simulink model "matrix6_drive"  (R2018b)
settings: Solver=VariableStepAuto  StartTime=0.0  StopTime=1  RelTol=1e-7
model workspace (MAT data in the model file):
  A1 = 0.212
  A2 = 0.0033
  AMP1 = 0.209333333333
  AMP2 = 0.0330526315789
  B1 = 0.311
  B2 = 0.0075
  C1 = 0.1
  C2 = 0.0084
  Ce1 = 0.27
  Ce2 = 0.12
  Cm1 = 0.36
  Cm2 = 0.12
  D1 = 0.1
  D2 = 0.001
  E1 = 0.1
  E2 = 0.001
  F1 = 0.1
  F2 = 0.001
  Jdrv1 = 7.5e-06
  Jdrv2 = 2.51e-06
  Kf1 = 0.1
  Kf2 = 0.1
  L1 = 0.032
  L2 = 0.0194
  R1 = 0.32
  R2 = 0.485
  RAMP = 0.209333333333
  T1 = 0.05
  T2 = 0.0001
  Tpwm = 6.25e-05
  Umax = 27
  Xc2 = 0
  Yc2 = 0.0148
  a = 0
  b = -2.09439510239
  c = 2.09439510239
  dt1 = 0.6
  dt2 = 0.6
  dx1 = 3.14
  dx2 = 1.57
  g = 9.81
  m2 = 1.13085
  omega1 = 1.005
  omega2 = 6.28
  poles = 8
libraries: simulink x1
(part 1 of 2)
settings Model: Creator=Sainquake  LastModifiedBy=Sainquake

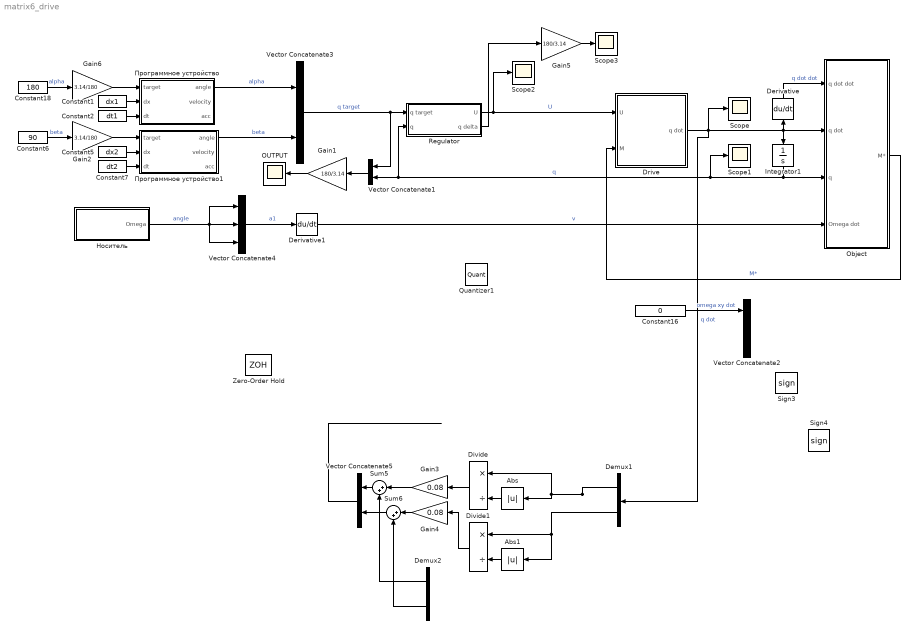
== system matrix6_drive ==
  Abs : Abs  ZeroCross=off
  Abs1 : Abs  ZeroCross=off
  Constant1 : Constant  Value=dx1
  Constant16 : Constant  Value=0
  Constant18 : Constant  Value=180
  Constant2 : Constant  Value=dt1
  Constant5 : Constant  Value=dx2
  Constant6 : Constant  Value=90
  Constant7 : Constant  Value=dt2
  Demux1 : Demux  Outputs=2
  Demux2 : Demux  Outputs=2
  Derivative : Derivative
  Derivative1 : Derivative
  Divide : Product  Inputs=*/
  Divide1 : Product  Inputs=*/
  Drive : Subsystem
  Gain1 : Gain  Gain=180/3.14
  Gain2 : Gain  Gain=3.14/180
  Gain3 : Gain  Gain=0.08
  Gain4 : Gain  Gain=0.08
  Gain5 : Gain  Gain=180/3.14
  Gain6 : Gain  Gain=3.14/180
  Integrator1 : Integrator
  OUTPUT : Scope
  Object : Subsystem
  Quantizer1 : Quantizer  QuantizationInterval=0.0003
  Regulator : Subsystem
  Scope{,1..3} (4 alike) : Scope
  Sign3 : Signum  ZeroCross=off
  Sign4 : Signum  ZeroCross=off
  Sum5 : Sum  Inputs=|++
  Sum6 : Sum  Inputs=|++
  Vector Concatenate1 : Concatenate
  Vector Concatenate2 : Concatenate  NumInputs=3
  Vector Concatenate3 : Concatenate
  Vector Concatenate4 : Concatenate  NumInputs=3
  Vector Concatenate5 : Concatenate
  Zero-Order Hold : ZeroOrderHold  SampleTime=Tpwm
  Носитель : Subsystem
  Программное устройство : Subsystem
  Программное устройство1 : Subsystem
  wires:
  Integrator1/1 -> Regulator/2(q), Vector Concatenate1/2, Scope1/1, Object/3("q ")  "q"
  ? -> Vector Concatenate2/3  "omega zy dot"
  ? -> Vector Concatenate2/2  "omega yy dot"
  Constant16/1 -> Vector Concatenate2/1  "omega xy dot"
  Программное устройство1/1(angle) -> Vector Concatenate3/2  "beta"
  Программное устройство/1(angle) -> Vector Concatenate3/1  "alpha"
  Drive/1(q dot) -> Demux1/1, Integrator1/1, Object/2(q dot), Derivative/1, Scope/1  "q dot"
  Object/1(M*) -> Drive/2(M)  "M*"
  Regulator/1("U ") -> Scope2/1, Drive/1(U)  "U"
  Divide/1 -> Gain3/1
  Divide1/1 -> Gain4/1
  Vector Concatenate5/1 -> ?
  Gain3/1 -> Sum5/1
  Demux2/1 -> Sum5/2
  Gain4/1 -> Sum6/1
  Demux2/2 -> Sum6/2
  Sum5/1 -> Vector Concatenate5/1
  Sum6/1 -> Vector Concatenate5/2
  Derivative/1 -> Object/1(q dot dot)  "q dot dot"
  Vector Concatenate3/1 -> Vector Concatenate1/1, Regulator/1(q target)  "q target"
  Vector Concatenate1/1 -> Gain1/1
  Gain1/1 -> OUTPUT/1
  Constant2/1 -> Программное устройство/3(dt)
  Gain6/1 -> Программное устройство/1(target)
  Constant1/1 -> Программное устройство/2("dx ")
  Constant18/1 -> Gain6/1  "alpha"
  Constant6/1 -> Gain2/1  "beta"
  Gain2/1 -> Программное устройство1/1(target)
  Constant7/1 -> Программное устройство1/3(dt)
  Constant5/1 -> Программное устройство1/2("dx ")
  Regulator/2(q delta) -> Gain5/1
  Gain5/1 -> Scope3/1
  Abs/1 -> Divide/2
  Demux1/1 -> Divide/1, Abs/1
  Abs1/1 -> Divide1/2
  Demux1/2 -> Abs1/1, Divide1/1
  Vector Concatenate4/1 -> Derivative1/1  "a1"
  Носитель/1(Omega) -> Vector Concatenate4/3, Vector Concatenate4/1, Vector Concatenate4/2  "angle"
  Derivative1/1 -> Object/4(Omega dot)  "v"

== system matrix6_drive/Drive ==
  U : Inport
  M : Inport  Port=2
  Demux : Demux  Outputs=2
  Demux1 : Demux  Outputs=2
  Scope : Scope
  Sum : Sum  Inputs=|+-
  Sum1 : Sum  Inputs=-+|
  Transfer Fcn : TransferFcn  Numerator=[Cm1]  Denominator=[L1 R1]
  Transfer Fcn1 : TransferFcn  Numerator=1  Denominator=[Cm1*Ce1]
  Transfer Fcn2 : TransferFcn  Numerator=[L1 R1]  Denominator=[0.0001 1]
  Transfer Fcn3 : TransferFcn  Numerator=[Cm2]  Denominator=[L2 R2]
  Transfer Fcn4 : TransferFcn  Numerator=1  Denominator=[Cm2*Ce2]
  Transfer Fcn5 : TransferFcn  Numerator=[L2 R2]  Denominator=[0.0001 1]
  Vector Concatenate6 : Concatenate
  Привод : Subsystem
  Привод1 : Subsystem
  q dot : Outport
  wires:
  Sum/1 -> Transfer Fcn2/1
  Transfer Fcn3/1 -> Sum1/2
  Demux1/2 -> Sum1/1
  Demux/1 -> Привод/1(U)
  Vector Concatenate6/1 -> q dot/1, Scope/1  "a1"
  Transfer Fcn/1 -> Sum/1
  Transfer Fcn5/1 -> Transfer Fcn4/1
  Transfer Fcn2/1 -> Transfer Fcn1/1
  Demux1/1 -> Привод/2(M load)
  Demux/2 -> Transfer Fcn3/1
  Sum1/1 -> Transfer Fcn5/1
  Transfer Fcn1/1 -> ?
  Transfer Fcn4/1 -> Vector Concatenate6/2
  U/1 -> Demux/1
  M/1 -> Demux1/1
  Привод/2(velocity) -> Vector Concatenate6/1
  Привод1/2(velocity) -> ?

== system matrix6_drive/Object ==
  q dot dot : Inport
  q dot : Inport  Port=2
  "q " : Inport  Port=3
  Omega dot : Inport  Port=4
  A(q) : Subsystem
  B(t,q) : Subsystem
  F(q,q dot) : Subsystem
  Integrator2 : Integrator
  Matrix Multiply1 : Product  Multiplication=Matrix(*)
  Matrix Multiply2 : Product  Multiplication=Matrix(*)
  Q*(t,q) : Subsystem
  Sum : Sum  Inputs=+++
  Sum1 : Sum  Inputs=+++
  W(t,q) : Subsystem
  M* : Outport
  wires:
  Integrator2/1 -> B(t,q)/1(omega), W(t,q)/1(Omega)
  Sum1/1 -> M*/1  "M*"
  A(q)/1(A) -> Matrix Multiply1/1
  q dot dot/1 -> Matrix Multiply1/2  "q dot dot"
  Omega dot/1 -> Integrator2/1, W(t,q)/2(Omega dot)  "a1"
  Sum/1 -> Sum1/1
  Matrix Multiply1/1 -> Sum/1
  Matrix Multiply2/1 -> Sum/2
  B(t,q)/1(B) -> Matrix Multiply2/1
  q dot/1 -> F(q,q dot)/1(q dot), Matrix Multiply2/2  "q dot"
  "q "/1 -> F(q,q dot)/2(q), B(t,q)/2(q), A(q)/1(q), Q*(t,q)/1(q), W(t,q)/3(q)  "q"
  W(t,q)/1(W) -> Sum1/2
  Q*(t,q)/1(Q) -> Sum1/3
  F(q,q dot)/1(F(q,q dot)) -> Sum/3

== system matrix6_drive/Regulator ==
  q target : Inport
  q : Inport  Port=2
  Demux : Demux  Outputs=2
  Demux3 : Demux  Outputs=2
  Gain2 : Gain  Gain=700
  Gain5 : Gain  Gain=300
  Saturation : Saturate  UpperLimit=27  LowerLimit=-27  ZeroCross=off
  Saturation1 : Saturate  UpperLimit=27  LowerLimit=-27  ZeroCross=off
  Sum2 : Sum  Inputs=|+-
  Sum3 : Sum  Inputs=|+-
  Transfer Fcn : TransferFcn  Numerator=[T1 1]  Denominator=[T2 1]
  Transfer Fcn1 : TransferFcn  Numerator=[0.05 1]  Denominator=[0.0005 1]
  Vector Concatenate1 : Concatenate
  Vector Concatenate2 : Concatenate
  "U " : Outport
  q delta : Outport  Port=2
  wires:
  Demux/1 -> Sum3/2
  Demux/2 -> Sum2/2
  Sum3/1 -> Vector Concatenate2/1, Gain2/1
  Transfer Fcn1/1 -> Vector Concatenate1/2
  Sum2/1 -> Vector Concatenate2/2, Gain5/1
  Transfer Fcn/1 -> Vector Concatenate1/1
  Demux3/2 -> Sum2/1
  Gain2/1 -> Transfer Fcn/1
  q target/1 -> Demux3/1  "q target"
  Gain5/1 -> Transfer Fcn1/1
  Demux3/1 -> Sum3/1
  q/1 -> Demux/1  "q"
  Vector Concatenate1/1 -> "U "/1  "U"
  Vector Concatenate2/1 -> q delta/1  "U"

== system matrix6_drive/Носитель ==
  Clock : Clock
  Gain : Gain  Gain=AMP1
  Gain1 : Gain  Gain=AMP2
  Gain2 : Gain  Gain=omega1
  Gain3 : Gain  Gain=omega2
  Ramp : simulink/Sources/Ramp  slope=RAMP  start=0  InitialOutput=0
  Sum1 : Sum  Inputs=+++
  Trigonometric Function : Trigonometry
  Trigonometric Function1 : Trigonometry
  Omega : Outport
  wires:
  Trigonometric Function/1 -> Gain/1
  Trigonometric Function1/1 -> Gain1/1
  Clock/1 -> Gain2/1, Gain3/1
  Gain2/1 -> Trigonometric Function/1
  Gain3/1 -> Trigonometric Function1/1
  Gain/1 -> Sum1/2
  Gain1/1 -> Sum1/3
  Sum1/1 -> Omega/1
  Ramp/1 -> Sum1/1

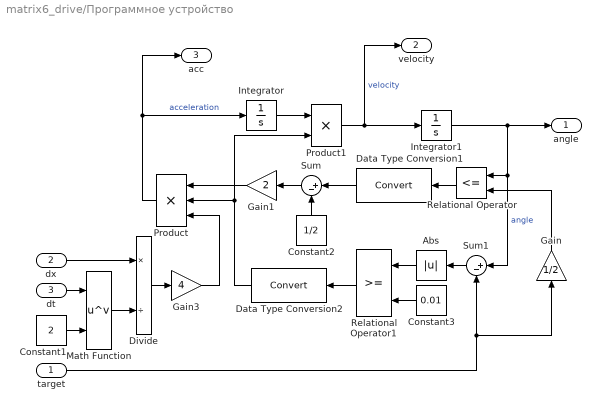
== system matrix6_drive/Программное устройство ==
  target : Inport
  "dx " : Inport  Port=2
  dt : Inport  Port=3
  Abs : Abs  ZeroCross=off
  Constant1 : Constant  Value=2
  Constant2 : Constant  Value=1/2
  Constant3 : Constant  Value=0.01
  Data Type Conversion1 : DataTypeConversion
  Data Type Conversion2 : DataTypeConversion
  Divide : Product  Inputs=*/
  Gain : Gain  Gain=1/2
  Gain1 : Gain  Gain=2
  Gain3 : Gain  Gain=4
  Integrator : Integrator
  Integrator1 : Integrator
  Math Function : Math  Operator=pow  SaturateOnIntegerOverflow=on
  Product : Product  Inputs=3
  Product1 : Product
  Relational Operator : RelationalOperator  Operator=<=  OutDataTypeStr=boolean  ZeroCross=off  RndMeth=Simplest
  Relational Operator1 : RelationalOperator  OutDataTypeStr=boolean  ZeroCross=off  RndMeth=Simplest
  Sum : Sum  Inputs=|+-
  Sum1 : Sum  Inputs=|+-
  angle : Outport
  velocity : Outport  Port=2
  acc : Outport  Port=3
  wires:
  "dx "/1 -> Divide/1
  Constant1/1 -> Math Function/2
  Gain3/1 -> Product/3
  Data Type Conversion1/1 -> Sum/1
  Sum/1 -> Gain1/1
  Product/1 -> Integrator/1, acc/1  "acceleration"
  Product1/1 -> Integrator1/1, velocity/1  "velocity"
  Abs/1 -> Relational Operator1/1
  Relational Operator1/1 -> Data Type Conversion2/1
  Sum1/1 -> Abs/1
  Data Type Conversion2/1 -> Product1/2, Product/2
  Divide/1 -> Gain3/1
  Constant2/1 -> Sum/2
  Integrator/1 -> Product1/1
  target/1 -> Gain/1, Sum1/2
  Math Function/1 -> Divide/2
  Gain/1 -> Relational Operator/2
  Gain1/1 -> Product/1
  Relational Operator/1 -> Data Type Conversion1/1
  dt/1 -> Math Function/1
  Constant3/1 -> Relational Operator1/2
  Integrator1/1 -> angle/1, Sum1/1, Relational Operator/1  "angle"

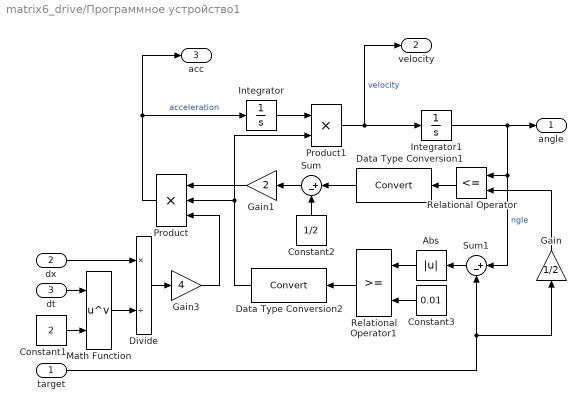
== system matrix6_drive/Программное устройство1 ==
  target : Inport
  "dx " : Inport  Port=2
  dt : Inport  Port=3
  Abs : Abs  ZeroCross=off
  Constant1 : Constant  Value=2
  Constant2 : Constant  Value=1/2
  Constant3 : Constant  Value=0.01
  Data Type Conversion1 : DataTypeConversion
  Data Type Conversion2 : DataTypeConversion
  Divide : Product  Inputs=*/
  Gain : Gain  Gain=1/2
  Gain1 : Gain  Gain=2
  Gain3 : Gain  Gain=4
  Integrator : Integrator
  Integrator1 : Integrator
  Math Function : Math  Operator=pow  SaturateOnIntegerOverflow=on
  Product : Product  Inputs=3
  Product1 : Product
  Relational Operator : RelationalOperator  Operator=<=  OutDataTypeStr=boolean  ZeroCross=off  RndMeth=Simplest
  Relational Operator1 : RelationalOperator  OutDataTypeStr=boolean  ZeroCross=off  RndMeth=Simplest
  Sum : Sum  Inputs=|+-
  Sum1 : Sum  Inputs=|+-
  angle : Outport
  velocity : Outport  Port=2
  acc : Outport  Port=3
  wires:
  "dx "/1 -> Divide/1
  Constant1/1 -> Math Function/2
  Gain3/1 -> Product/3
  Data Type Conversion1/1 -> Sum/1
  Sum/1 -> Gain1/1
  Product/1 -> Integrator/1, acc/1  "acceleration"
  Product1/1 -> Integrator1/1, velocity/1  "velocity"
  Abs/1 -> Relational Operator1/1
  Relational Operator1/1 -> Data Type Conversion2/1
  Sum1/1 -> Abs/1
  Data Type Conversion2/1 -> Product1/2, Product/2
  Divide/1 -> Gain3/1
  Constant2/1 -> Sum/2
  Integrator/1 -> Product1/1
  target/1 -> Gain/1, Sum1/2
  Math Function/1 -> Divide/2
  Gain/1 -> Relational Operator/2
  Gain1/1 -> Product/1
  Relational Operator/1 -> Data Type Conversion1/1
  dt/1 -> Math Function/1
  Constant3/1 -> Relational Operator1/2
  Integrator1/1 -> angle/1, Sum1/1, Relational Operator/1  "ngle"

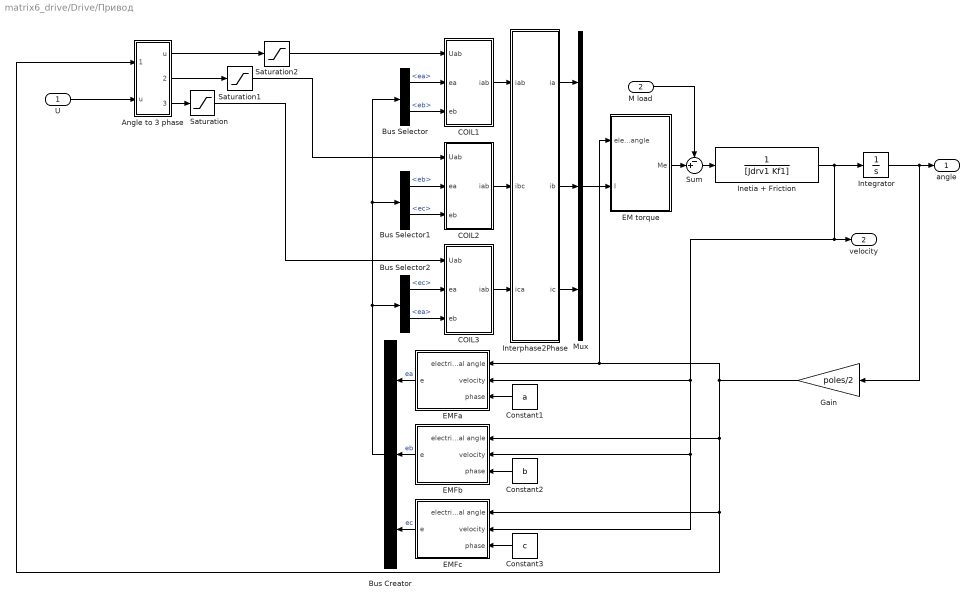
== system matrix6_drive/Drive/Привод ==
  U : Inport
  M load : Inport  Port=2
  Angle to 3 phase : Subsystem
  Bus Creator : BusCreator  Inputs=3
  Bus Selector : BusSelector  OutputSignals=ea,eb
  Bus Selector1 : BusSelector  OutputSignals=eb,ec
  Bus Selector2 : BusSelector  OutputSignals=ec,ea
  COIL1 : Subsystem
  "COIL2 " : Subsystem
  COIL3 : Subsystem
  Constant1 : Constant  Value=a
  Constant2 : Constant  Value=b
  Constant3 : Constant  Value=c
  EM torque : Subsystem
  EMFa : Subsystem
  EMFb : Subsystem
  EMFc : Subsystem
  Gain : Gain  Gain=poles/2
  Inetia + Friction : TransferFcn  Denominator=[Jdrv1 Kf1]
  Integrator : Integrator
  Interphase2Phase : Subsystem
  Mux : Mux  Inputs=3
  Saturation : Saturate  UpperLimit=Umax  LowerLimit=0  ZeroCross=off
  Saturation1 : Saturate  UpperLimit=Umax  LowerLimit=0  ZeroCross=off
  Saturation2 : Saturate  UpperLimit=Umax  LowerLimit=0  ZeroCross=off
  Sum : Sum  Inputs=-+|
  angle : Outport
  velocity : Outport  Port=2
  wires:
  M load/1 -> Sum/1
  Bus Creator/1 -> Bus Selector/1, Bus Selector1/1, Bus Selector2/1
  COIL1/1(iab) -> Interphase2Phase/1(iab)
  Interphase2Phase/1(ia) -> Mux/1
  Bus Selector2/2 -> COIL3/3(eb)  "<ea>"
  Gain/1 -> Angle to 3 phase/1(target), EMFc/1(electrical angle), EMFb/1(electrical angle), EM torque/1(electrical angle), EMFa/1(electrical angle)
  Bus Selector2/1 -> COIL3/2("ea ")  "<ec>"
  Bus Selector1/1 -> "COIL2 "/2("ea ")  "<eb>"
  Bus Selector1/2 -> "COIL2 "/3(eb)  "<ec>"
  Mux/1 -> EM torque/2(I)
  Bus Selector/2 -> COIL1/3(eb)  "<eb>"
  Bus Selector/1 -> COIL1/2("ea ")  "<ea>"
  Sum/1 -> Inetia + Friction/1
  Constant2/1 -> EMFb/3(phase)
  Constant3/1 -> EMFc/3(phase)
  Constant1/1 -> EMFa/3(phase)
  Inetia + Friction/1 -> Integrator/1, velocity/1, EMFc/2(velocity), EMFb/2(velocity), EMFa/2(velocity)
  EMFa/1(e) -> Bus Creator/1  "ea"
  EMFc/1(e) -> Bus Creator/3  "ec"
  EM torque/1(Me) -> Sum/2
  Interphase2Phase/3(ic) -> Mux/3
  "COIL2 "/1(iab) -> Interphase2Phase/2("ibc ")
  Angle to 3 phase/1("u ") -> Saturation2/1
  EMFb/1(e) -> Bus Creator/2  "eb"
  Angle to 3 phase/3(u 2) -> Saturation/1
  Angle to 3 phase/2(u 1) -> Saturation1/1
  Interphase2Phase/2(ib) -> Mux/2
  COIL3/1(iab) -> Interphase2Phase/3(ica)
  U/1 -> Angle to 3 phase/2(u)
  Integrator/1 -> Gain/1, angle/1
  Saturation2/1 -> COIL1/1(Uab)
  Saturation1/1 -> "COIL2 "/1(Uab)
  Saturation/1 -> COIL3/1(Uab)

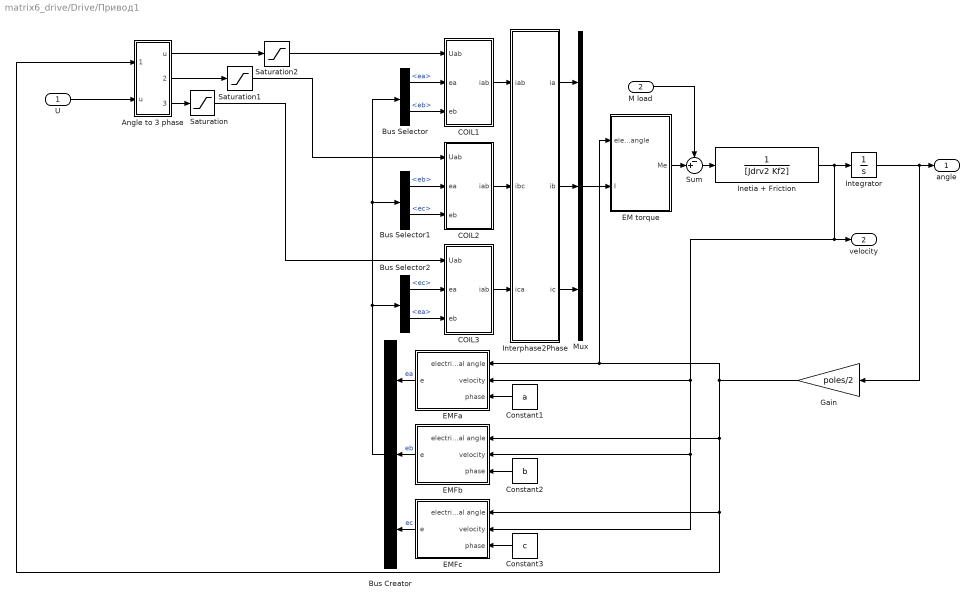
== system matrix6_drive/Drive/Привод1 ==
  U : Inport
  M load : Inport  Port=2
  Angle to 3 phase : Subsystem
  Bus Creator : BusCreator  Inputs=3
  Bus Selector : BusSelector  OutputSignals=ea,eb
  Bus Selector1 : BusSelector  OutputSignals=eb,ec
  Bus Selector2 : BusSelector  OutputSignals=ec,ea
  COIL1 : Subsystem
  "COIL2 " : Subsystem
  COIL3 : Subsystem
  Constant1 : Constant  Value=a
  Constant2 : Constant  Value=b
  Constant3 : Constant  Value=c
  EM torque : Subsystem
  EMFa : Subsystem
  EMFb : Subsystem
  EMFc : Subsystem
  Gain : Gain  Gain=poles/2
  Inetia + Friction : TransferFcn  Denominator=[Jdrv2 Kf2]
  Integrator : Integrator
  Interphase2Phase : Subsystem
  Mux : Mux  Inputs=3
  Saturation : Saturate  UpperLimit=Umax  LowerLimit=0  ZeroCross=off
  Saturation1 : Saturate  UpperLimit=Umax  LowerLimit=0  ZeroCross=off
  Saturation2 : Saturate  UpperLimit=Umax  LowerLimit=0  ZeroCross=off
  Sum : Sum  Inputs=-+|
  angle : Outport
  velocity : Outport  Port=2
  wires:
  Saturation/1 -> COIL3/1(Uab)
  Saturation1/1 -> "COIL2 "/1(Uab)
  Saturation2/1 -> COIL1/1(Uab)
  Integrator/1 -> Gain/1, angle/1
  U/1 -> Angle to 3 phase/2(u)
  COIL3/1(iab) -> Interphase2Phase/3(ica)
  Interphase2Phase/2(ib) -> Mux/2
  Angle to 3 phase/2(u 1) -> Saturation1/1
  Angle to 3 phase/3(u 2) -> Saturation/1
  EMFb/1(e) -> Bus Creator/2  "eb"
  Angle to 3 phase/1("u ") -> Saturation2/1
  "COIL2 "/1(iab) -> Interphase2Phase/2("ibc ")
  Interphase2Phase/3(ic) -> Mux/3
  EM torque/1(Me) -> Sum/2
  EMFc/1(e) -> Bus Creator/3  "ec"
  EMFa/1(e) -> Bus Creator/1  "ea"
  Inetia + Friction/1 -> Integrator/1, EMFa/2(velocity), EMFb/2(velocity), EMFc/2(velocity), velocity/1
  Constant1/1 -> EMFa/3(phase)
  Constant3/1 -> EMFc/3(phase)
  Constant2/1 -> EMFb/3(phase)
  Sum/1 -> Inetia + Friction/1
  Bus Selector/1 -> COIL1/2("ea ")  "<ea>"
  Bus Selector/2 -> COIL1/3(eb)  "<eb>"
  Mux/1 -> EM torque/2(I)
  Bus Selector1/2 -> "COIL2 "/3(eb)  "<ec>"
  Bus Selector1/1 -> "COIL2 "/2("ea ")  "<eb>"
  Bus Selector2/1 -> COIL3/2("ea ")  "<ec>"
  Gain/1 -> EMFa/1(electrical angle), EM torque/1(electrical angle), EMFb/1(electrical angle), EMFc/1(electrical angle), Angle to 3 phase/1(target)
  Bus Selector2/2 -> COIL3/3(eb)  "<ea>"
  Interphase2Phase/1(ia) -> Mux/1
  COIL1/1(iab) -> Interphase2Phase/1(iab)
  Bus Creator/1 -> Bus Selector2/1, Bus Selector1/1, Bus Selector/1
  M load/1 -> Sum/1

== system matrix6_drive/Object/A(q) ==
  q : Inport
  B(beta) : Subsystem
  Constant10 : Constant  Value=C2
  Constant7 : Constant  Value=B1
  D(beta) : Subsystem
  Demux : Demux  Outputs=2
  Display5 : Display
  Gain : Gain  Gain=-1
  Sum : Sum  Inputs=|++
  Vector Concatenate1 : Concatenate
  Vector Concatenate2 : Concatenate
  Vector Concatenate6 : Concatenate  Mode=Multidimensional array  ConcatenateDimension=2
  A : Outport
  wires:
  q/1 -> Demux/1
  Constant7/1 -> Sum/2
  Vector Concatenate2/1 -> Vector Concatenate6/2  "a2"
  Sum/1 -> Vector Concatenate1/1  "a11"
  Constant10/1 -> Vector Concatenate2/2  "a22"
  Vector Concatenate1/1 -> Vector Concatenate6/1  "a1"
  B(beta)/1(B) -> Sum/1
  D(beta)/1(D) -> Gain/1
  Vector Concatenate6/1 -> A/1, Display5/1  "A"
  Gain/1 -> Vector Concatenate1/2, Vector Concatenate2/1  "a12"
  Demux/2 -> B(beta)/1(beta), D(beta)/1(beta)

== system matrix6_drive/Object/B(t,q) ==
  omega : Inport
  q : Inport  Port=2
  Constant : Constant  Value=0
  Gain : Gain  Gain=-1
  Vector Concatenate3 : Concatenate
  Vector Concatenate4 : Concatenate
  Vector Concatenate5 : Concatenate  Mode=Multidimensional array  ConcatenateDimension=2
  b(t,alpha,beta) : Subsystem
  B : Outport
  wires:
  Vector Concatenate3/1 -> Vector Concatenate5/1  "a1"
  Vector Concatenate5/1 -> B/1  "A"
  Vector Concatenate4/1 -> Vector Concatenate5/2  "a2"
  b(t,alpha,beta)/1(b) -> Vector Concatenate3/2, Gain/1
  Gain/1 -> Vector Concatenate4/1
  Constant/1 -> Vector Concatenate4/2, Vector Concatenate3/1
  omega/1 -> b(t,alpha,beta)/1(omega)
  q/1 -> b(t,alpha,beta)/2(q)

== system matrix6_drive/Object/F(q,q dot) ==
  q dot : Inport
  q : Inport  Port=2
  Constant : Constant  Value=2
  Constant1 : Constant  Value=2
  Demux : Demux  Outputs=2
  Demux1 : Demux  Outputs=2
  E(beta) : Subsystem
  F(alpha,beta) : Subsystem
  F(beta) : Subsystem
  Gain : Gain  Gain=2
  Math Function : Math  Operator=pow  SaturateOnIntegerOverflow=on
  Math Function1 : Math  Operator=pow  SaturateOnIntegerOverflow=on
  Product : Product  Inputs=3
  Product1 : Product
  Product2 : Product
  Sum : Sum  Inputs=|--
  Vector Concatenate : Concatenate
  F(q,q dot) : Outport
  wires:
  q dot/1 -> Demux/1
  Product/1 -> Gain/1
  Demux/2 -> Product/2, Math Function/1  "beta dot"
  F(alpha,beta)/1(F(q)) -> Product/3
  q/1 -> Demux1/1, F(alpha,beta)/1(q)
  Constant/1 -> Math Function/2
  Math Function/1 -> Product1/1
  E(beta)/1(E) -> Product1/2
  Demux1/2 -> E(beta)/1(beta), F(beta)/1(beta)
  Gain/1 -> Sum/1
  Product1/1 -> Sum/2
  Constant1/1 -> Math Function1/2
  Demux/1 -> Product/1, Math Function1/1  "alpha dot"
  Math Function1/1 -> Product2/2
  F(beta)/1(F) -> Product2/1
  Product2/1 -> Vector Concatenate/2
  Sum/1 -> Vector Concatenate/1
  Vector Concatenate/1 -> F(q,q dot)/1

== system matrix6_drive/Object/Q*(t,q) ==
  q : Inport
  Constant : Constant  Value=0
  Constant1 : Constant  Value=m2
  Constant2 : Constant  Value=Xc2
  Constant3 : Constant  Value=Yc2
  Demux : Demux  Outputs=2
  Gain : Gain  Gain=g
  Product : Product
  Product1 : Product
  Product2 : Product
  Sum : Sum  Inputs=+-
  Trigonometric Function : Trigonometry  Operator=cos
  Trigonometric Function1 : Trigonometry
  Vector Concatenate1 : Concatenate
  Q : Outport
  wires:
  Vector Concatenate1/1 -> Q/1  "q"
  Constant/1 -> Vector Concatenate1/1
  Product/1 -> Vector Concatenate1/2
  Gain/1 -> Product/1
  Constant1/1 -> Gain/1
  q/1 -> Demux/1
  Trigonometric Function/1 -> Product1/1
  Constant2/1 -> Product1/2
  Product1/1 -> Sum/1
  Constant3/1 -> Product2/2
  Demux/2 -> Trigonometric Function1/1, Trigonometric Function/1  "beta"
  Product2/1 -> Sum/2
  Trigonometric Function1/1 -> Product2/1
  Sum/1 -> Product/2

== system matrix6_drive/Object/W(t,q) ==
  Omega : Inport
  Omega dot : Inport  Port=2
  q : Inport  Port=3
  Vector Concatenate : Concatenate
  "w alpha (t, q) " : Subsystem
  "w beta (t, q)" : Subsystem
  W : Outport
  wires:
  Omega/1 -> "w beta (t, q)"/1(Omega), "w alpha (t, q) "/1(Omega)
  Omega dot/1 -> "w beta (t, q)"/2(Omega dot), "w alpha (t, q) "/2(Omega dot)
  q/1 -> "w beta (t, q)"/3(q), "w alpha (t, q) "/3(q)
  "w alpha (t, q) "/1(w alpha) -> Vector Concatenate/1
  "w beta (t, q)"/1(w alpha) -> Vector Concatenate/2
  Vector Concatenate/1 -> W/1

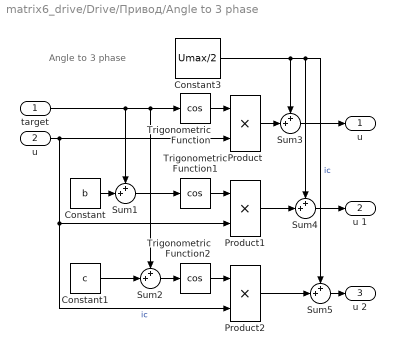
== system matrix6_drive/Drive/Привод/Angle to 3 phase ==
  note: Angle to 3 phase
  target : Inport
  u : Inport  Port=2
  Constant : Constant  Value=b
  Constant1 : Constant  Value=c
  Constant3 : Constant  Value=Umax/2
  Product : Product
  Product1 : Product
  Product2 : Product
  Sum{1..5} (5 alike) : Sum  Inputs=++|
  Trigonometric Function : Trigonometry  Operator=cos
  Trigonometric Function1 : Trigonometry  Operator=cos
  Trigonometric Function2 : Trigonometry  Operator=cos
  "u " : Outport
  u 1 : Outport  Port=2
  u 2 : Outport  Port=3
  wires:
  Sum3/1 -> "u "/1
  target/1 -> Sum2/1, Trigonometric Function/1, Sum1/1
  Trigonometric Function2/1 -> Product2/1
  Sum2/1 -> Trigonometric Function2/1
  Trigonometric Function1/1 -> Product1/1
  u/1 -> Product/2, Product2/2, Product1/2  "ic"
  Constant1/1 -> Sum2/2
  Sum1/1 -> Trigonometric Function1/1
  Constant/1 -> Sum1/2
  Trigonometric Function/1 -> Product/1
  Constant3/1 -> Sum5/1, Sum4/1, Sum3/1  "ic"
  Product/1 -> Sum3/2
  Product1/1 -> Sum4/2
  Product2/1 -> Sum5/2
  Sum5/1 -> u 2/1
  Sum4/1 -> u 1/1

== system matrix6_drive/Drive/Привод/COIL1 ==
  note: COILx
  Uab : Inport
  "ea " : Inport  Port=2
  eb : Inport  Port=3
  Sum : Sum  Inputs=|+-
  Sum1 : Sum  Inputs=|+-
  Transfer Fcn : TransferFcn  Denominator=[L1 R1]
  iab : Outport
  wires:
  Uab/1 -> Sum/1
  Transfer Fcn/1 -> iab/1
  Sum/1 -> Transfer Fcn/1
  "ea "/1 -> Sum1/1
  eb/1 -> Sum1/2
  Sum1/1 -> Sum/2

== system matrix6_drive/Drive/Привод/COIL2  ==
  Uab : Inport
  "ea " : Inport  Port=2
  eb : Inport  Port=3
  Sum : Sum  Inputs=|+-
  Sum1 : Sum  Inputs=|+-
  Transfer Fcn : TransferFcn  Denominator=[L1 R1]
  iab : Outport
  wires:
  Uab/1 -> Sum/1
  Transfer Fcn/1 -> iab/1
  Sum/1 -> Transfer Fcn/1
  "ea "/1 -> Sum1/1
  eb/1 -> Sum1/2
  Sum1/1 -> Sum/2

== system matrix6_drive/Drive/Привод/COIL3 ==
  Uab : Inport
  "ea " : Inport  Port=2
  eb : Inport  Port=3
  Sum : Sum  Inputs=|+-
  Sum1 : Sum  Inputs=|+-
  Transfer Fcn : TransferFcn  Denominator=[L1 R1]
  iab : Outport
  wires:
  Uab/1 -> Sum/1
  Transfer Fcn/1 -> iab/1
  Sum/1 -> Transfer Fcn/1
  "ea "/1 -> Sum1/1
  eb/1 -> Sum1/2
  Sum1/1 -> Sum/2

== system matrix6_drive/Drive/Привод/EM torque ==
  note: Electromagnetic Torque
  electrical angle : Inport
  I : Inport  Port=2
  Constant2 : Constant  Value=a
  Constant3 : Constant  Value=b
  Constant4 : Constant  Value=c
  Demux : Demux  Outputs=3
  Gain : Gain  Gain=Cm1
  Product3 : Product
  Product4 : Product
  Product5 : Product
  Subsystem : Subsystem
  Subsystem1 : Subsystem
  Subsystem2 : Subsystem
  Sum : Sum  Inputs=+++
  Me : Outport
  wires:
  Sum/1 -> Gain/1
  Gain/1 -> Me/1
  I/1 -> Demux/1
  Constant2/1 -> Subsystem/2(phase)
  electrical angle/1 -> Subsystem2/1(electrical angle), Subsystem1/1(electrical angle), Subsystem/1(electrical angle)
  Constant3/1 -> Subsystem1/2(phase)
  Constant4/1 -> Subsystem2/2(phase)
  Demux/1 -> Product3/2  "ia"
  Subsystem/1(Out1) -> Product3/1
  Demux/2 -> Product4/2  "ib"
  Demux/3 -> Product5/2  "ic"
  Subsystem1/1(Out1) -> Product4/1
  Subsystem2/1(Out1) -> Product5/1
  Product4/1 -> Sum/2
  Product3/1 -> Sum/1
  Product5/1 -> Sum/3

== system matrix6_drive/Drive/Привод/EMFa ==
  note: EMF
  electrical angle : Inport
  velocity : Inport  Port=2
  phase : Inport  Port=3
  Gain : Gain  Gain=Ce1
  Product1 : Product
  Subsystem : Subsystem
  e : Outport
  wires:
  Gain/1 -> Product1/2
  Product1/1 -> e/1
  velocity/1 -> Gain/1
  phase/1 -> Subsystem/2(phase)
  electrical angle/1 -> Subsystem/1(electrical angle)
  Subsystem/1(Out1) -> Product1/1

== system matrix6_drive/Drive/Привод/EMFb ==
  electrical angle : Inport
  velocity : Inport  Port=2
  phase : Inport  Port=3
  Gain : Gain  Gain=Ce1
  Product1 : Product
  Sum1 : Sum  Inputs=++|
  Trigonometric Function1 : Trigonometry  Operator=cos
  e : Outport
  wires:
  Trigonometric Function1/1 -> Product1/1
  Gain/1 -> Product1/2
  Sum1/1 -> Trigonometric Function1/1
  phase/1 -> Sum1/2
  electrical angle/1 -> Sum1/1
  Product1/1 -> e/1
  velocity/1 -> Gain/1

== system matrix6_drive/Drive/Привод/EMFc ==
  electrical angle : Inport
  velocity : Inport  Port=2
  phase : Inport  Port=3
  Gain : Gain  Gain=Ce1
  Product1 : Product
  Sum1 : Sum  Inputs=++|
  Trigonometric Function1 : Trigonometry  Operator=cos
  e : Outport
  wires:
  Trigonometric Function1/1 -> Product1/1
  Gain/1 -> Product1/2
  Sum1/1 -> Trigonometric Function1/1
  phase/1 -> Sum1/2
  electrical angle/1 -> Sum1/1
  Product1/1 -> e/1
  velocity/1 -> Gain/1

== system matrix6_drive/Drive/Привод/Interphase2Phase ==
  note: Interphase to phase currents
  iab : Inport
  "ibc " : Inport  Port=2
  ica : Inport  Port=3
  Gain : Gain  Gain=1/2
  Gain1 : Gain  Gain=1/2
  Gain2 : Gain  Gain=1/2
  Sum : Sum  Inputs=+--
  Sum1 : Sum  Inputs=+--
  Sum2 : Sum  Inputs=+--
  ia : Outport
  ib : Outport  Port=2
  ic : Outport  Port=3
  wires:
  Gain/1 -> ia/1
  Gain1/1 -> ib/1
  Gain2/1 -> ic/1
  iab/1 -> Sum2/3, Sum1/3, Sum/1
  "ibc "/1 -> Sum2/2, Sum1/1, Sum/2
  ica/1 -> Sum/3, Sum2/1, Sum1/2
  Sum/1 -> Gain/1
  Sum1/1 -> Gain1/1
  Sum2/1 -> Gain2/1

== system matrix6_drive/Drive/Привод1/Angle to 3 phase ==
  note: Angle to 3 phase
  target : Inport
  u : Inport  Port=2
  Constant : Constant  Value=b
  Constant1 : Constant  Value=c
  Constant3 : Constant  Value=Umax/2
  Product : Product
  Product1 : Product
  Product2 : Product
  Sum{1..5} (5 alike) : Sum  Inputs=++|
  Trigonometric Function : Trigonometry  Operator=cos
  Trigonometric Function1 : Trigonometry  Operator=cos
  Trigonometric Function2 : Trigonometry  Operator=cos
  "u " : Outport
  u 1 : Outport  Port=2
  u 2 : Outport  Port=3
  wires:
  Sum4/1 -> u 1/1
  Sum5/1 -> u 2/1
  Product2/1 -> Sum5/2
  Product1/1 -> Sum4/2
  Product/1 -> Sum3/2
  Constant3/1 -> Sum3/1, Sum4/1, Sum5/1  "ic"
  Trigonometric Function/1 -> Product/1
  Constant/1 -> Sum1/2
  Sum1/1 -> Trigonometric Function1/1
  Constant1/1 -> Sum2/2
  u/1 -> Product1/2, Product2/2, Product/2  "ic"
  Trigonometric Function1/1 -> Product1/1
  Sum2/1 -> Trigonometric Function2/1
  Trigonometric Function2/1 -> Product2/1
  target/1 -> Sum1/1, Trigonometric Function/1, Sum2/1
  Sum3/1 -> "u "/1

== system matrix6_drive/Drive/Привод1/COIL1 ==
  note: COILx
  Uab : Inport
  "ea " : Inport  Port=2
  eb : Inport  Port=3
  Sum : Sum  Inputs=|+-
  Sum1 : Sum  Inputs=|+-
  Transfer Fcn : TransferFcn  Denominator=[L2 R2]
  iab : Outport
  wires:
  Sum1/1 -> Sum/2
  eb/1 -> Sum1/2
  "ea "/1 -> Sum1/1
  Sum/1 -> Transfer Fcn/1
  Transfer Fcn/1 -> iab/1
  Uab/1 -> Sum/1

== system matrix6_drive/Drive/Привод1/COIL2  ==
  Uab : Inport
  "ea " : Inport  Port=2
  eb : Inport  Port=3
  Sum : Sum  Inputs=|+-
  Sum1 : Sum  Inputs=|+-
  Transfer Fcn : TransferFcn  Denominator=[L2 R2]
  iab : Outport
  wires:
  Sum1/1 -> Sum/2
  eb/1 -> Sum1/2
  "ea "/1 -> Sum1/1
  Sum/1 -> Transfer Fcn/1
  Transfer Fcn/1 -> iab/1
  Uab/1 -> Sum/1

== system matrix6_drive/Drive/Привод1/COIL3 ==
  Uab : Inport
  "ea " : Inport  Port=2
  eb : Inport  Port=3
  Sum : Sum  Inputs=|+-
  Sum1 : Sum  Inputs=|+-
  Transfer Fcn : TransferFcn  Denominator=[L2 R2]
  iab : Outport
  wires:
  Sum1/1 -> Sum/2
  eb/1 -> Sum1/2
  "ea "/1 -> Sum1/1
  Sum/1 -> Transfer Fcn/1
  Transfer Fcn/1 -> iab/1
  Uab/1 -> Sum/1

== system matrix6_drive/Drive/Привод1/EM torque ==
  note: Electromagnetic Torque
  electrical angle : Inport
  I : Inport  Port=2
  Constant2 : Constant  Value=a
  Constant3 : Constant  Value=b
  Constant4 : Constant  Value=c
  Demux : Demux  Outputs=3
  Gain : Gain  Gain=Cm2
  Product3 : Product
  Product4 : Product
  Product5 : Product
  Subsystem : Subsystem
  Subsystem1 : Subsystem
  Subsystem2 : Subsystem
  Sum : Sum  Inputs=+++
  Me : Outport
  wires:
  Product5/1 -> Sum/3
  Product3/1 -> Sum/1
  Product4/1 -> Sum/2
  Subsystem2/1(Out1) -> Product5/1
  Subsystem1/1(Out1) -> Product4/1
  Demux/3 -> Product5/2  "ic"
  Demux/2 -> Product4/2  "ib"
  Subsystem/1(Out1) -> Product3/1
  Demux/1 -> Product3/2  "ia"
  Constant4/1 -> Subsystem2/2(phase)
  Constant3/1 -> Subsystem1/2(phase)
  electrical angle/1 -> Subsystem/1(electrical angle), Subsystem1/1(electrical angle), Subsystem2/1(electrical angle)
  Constant2/1 -> Subsystem/2(phase)
  I/1 -> Demux/1
  Gain/1 -> Me/1
  Sum/1 -> Gain/1

== system matrix6_drive/Drive/Привод1/EMFa ==
  note: EMF
  electrical angle : Inport
  velocity : Inport  Port=2
  phase : Inport  Port=3
  Gain : Gain  Gain=Ce2
  Product1 : Product
  Subsystem : Subsystem
  e : Outport
  wires:
  Subsystem/1(Out1) -> Product1/1
  electrical angle/1 -> Subsystem/1(electrical angle)
  phase/1 -> Subsystem/2(phase)
  velocity/1 -> Gain/1
  Product1/1 -> e/1
  Gain/1 -> Product1/2

== system matrix6_drive/Drive/Привод1/EMFb ==
  electrical angle : Inport
  velocity : Inport  Port=2
  phase : Inport  Port=3
  Gain : Gain  Gain=Ce2
  Product1 : Product
  Sum1 : Sum  Inputs=++|
  Trigonometric Function1 : Trigonometry  Operator=cos
  e : Outport
  wires:
  velocity/1 -> Gain/1
  Product1/1 -> e/1
  electrical angle/1 -> Sum1/1
  phase/1 -> Sum1/2
  Sum1/1 -> Trigonometric Function1/1
  Gain/1 -> Product1/2
  Trigonometric Function1/1 -> Product1/1

== system matrix6_drive/Drive/Привод1/EMFc ==
  electrical angle : Inport
  velocity : Inport  Port=2
  phase : Inport  Port=3
  Gain : Gain  Gain=Ce2
  Product1 : Product
  Sum1 : Sum  Inputs=++|
  Trigonometric Function1 : Trigonometry  Operator=cos
  e : Outport
  wires:
  velocity/1 -> Gain/1
  Product1/1 -> e/1
  electrical angle/1 -> Sum1/1
  phase/1 -> Sum1/2
  Sum1/1 -> Trigonometric Function1/1
  Gain/1 -> Product1/2
  Trigonometric Function1/1 -> Product1/1

== system matrix6_drive/Drive/Привод1/Interphase2Phase ==
  note: Interphase to phase currents
  iab : Inport
  "ibc " : Inport  Port=2
  ica : Inport  Port=3
  Gain : Gain  Gain=1/2
  Gain1 : Gain  Gain=1/2
  Gain2 : Gain  Gain=1/2
  Sum : Sum  Inputs=+--
  Sum1 : Sum  Inputs=+--
  Sum2 : Sum  Inputs=+--
  ia : Outport
  ib : Outport  Port=2
  ic : Outport  Port=3
  wires:
  Sum2/1 -> Gain2/1
  Sum1/1 -> Gain1/1
  Sum/1 -> Gain/1
  ica/1 -> Sum1/2, Sum2/1, Sum/3
  "ibc "/1 -> Sum/2, Sum1/1, Sum2/2
  iab/1 -> Sum/1, Sum1/3, Sum2/3
  Gain2/1 -> ic/1
  Gain1/1 -> ib/1
  Gain/1 -> ia/1

== system matrix6_drive/Object/A(q)/B(beta) ==
  beta : Inport
  Constant3 : Constant  Value=2
  Constant4 : Constant  Value=2
  Gain : Gain  Gain=B2
  Gain1 : Gain  Gain=A2
  Gain2 : Gain  Gain=F2
  Gain3 : Gain  Gain=2
  Math Function : Math  Operator=pow  SaturateOnIntegerOverflow=on
  Math Function1 : Math  Operator=pow  SaturateOnIntegerOverflow=on
  Sum : Sum  Inputs=++-
  Trigonometric Function : Trigonometry  Operator=cos
  Trigonometric Function1 : Trigonometry
  Trigonometric Function2 : Trigonometry
  B : Outport
  wires:
  beta/1 -> Gain3/1, Trigonometric Function1/1, Trigonometric Function/1
  Constant3/1 -> Math Function/2
  Trigonometric Function/1 -> Math Function/1
  Math Function/1 -> Gain/1
  Trigonometric Function1/1 -> Math Function1/1
  Math Function1/1 -> Gain1/1
  Constant4/1 -> Math Function1/2
  Trigonometric Function2/1 -> Gain2/1
  Gain3/1 -> Trigonometric Function2/1
  Gain1/1 -> Sum/2
  Gain/1 -> Sum/1
  Gain2/1 -> Sum/3
  Sum/1 -> B/1

== system matrix6_drive/Object/A(q)/D(beta) ==
  beta : Inport
  Gain : Gain  Gain=D2
  Gain2 : Gain  Gain=E2
  Sum : Sum
  Trigonometric Function : Trigonometry  Operator=cos
  Trigonometric Function2 : Trigonometry
  D : Outport
  wires:
  Trigonometric Function/1 -> Gain/1
  Trigonometric Function2/1 -> Gain2/1
  beta/1 -> Trigonometric Function2/1, Trigonometric Function/1
  Gain/1 -> Sum/1
  Sum/1 -> D/1
  Gain2/1 -> Sum/2

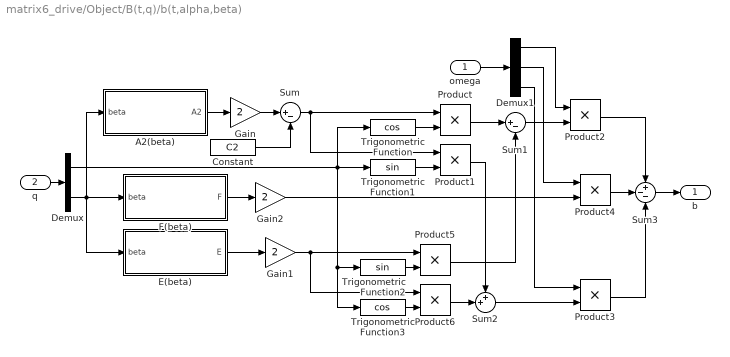
== system matrix6_drive/Object/B(t,q)/b(t,alpha,beta) ==
  omega : Inport
  q : Inport  Port=2
  A2(beta) : Subsystem
  Constant : Constant  Value=C2
  Demux : Demux  Outputs=2
  Demux1 : Demux  Outputs=3
  E(beta) : Subsystem
  F(beta) : Subsystem
  Gain : Gain  Gain=2
  Gain1 : Gain  Gain=2
  Gain2 : Gain  Gain=2
  Product{,1..6} (7 alike) : Product
  Sum : Sum  Inputs=|+-
  Sum1 : Sum  Inputs=|+-
  Sum2 : Sum  Inputs=++|
  Sum3 : Sum  Inputs=+--
  Trigonometric Function : Trigonometry  Operator=cos
  Trigonometric Function1 : Trigonometry
  Trigonometric Function2 : Trigonometry
  Trigonometric Function3 : Trigonometry  Operator=cos
  b : Outport
  wires:
  q/1 -> Demux/1
  omega/1 -> Demux1/1
  A2(beta)/1(A2) -> Gain/1
  Constant/1 -> Sum/2
  Gain/1 -> Sum/1
  Sum/1 -> Product1/1, Product/1
  Trigonometric Function/1 -> Product/2
  Demux/1 -> Trigonometric Function3/1, Trigonometric Function2/1, Trigonometric Function1/1, Trigonometric Function/1
  Trigonometric Function1/1 -> Product1/2
  Demux1/1 -> Product2/1
  Trigonometric Function3/1 -> Product6/2
  Trigonometric Function2/1 -> Product5/2
  E(beta)/1(E) -> Gain1/1
  Gain1/1 -> Product6/1, Product5/1
  Demux/2 -> E(beta)/1(beta), A2(beta)/1(beta), F(beta)/1(beta)
  Product/1 -> Sum1/1
  Product5/1 -> Sum1/2
  Product6/1 -> Sum2/2
  Product1/1 -> Sum2/1
  Sum1/1 -> Product2/2
  F(beta)/1(F) -> Gain2/1
  Gain2/1 -> Product4/2
  Demux1/2 -> Product4/1
  Demux1/3 -> Product3/1
  Sum2/1 -> Product3/2
  Product2/1 -> Sum3/1
  Product4/1 -> Sum3/2
  Product3/1 -> Sum3/3
  Sum3/1 -> b/1

== system matrix6_drive/Object/F(q,q dot)/E(beta) ==
  beta : Inport
  Gain : Gain  Gain=E2
  Gain2 : Gain  Gain=D2
  Sum : Sum  Inputs=+-
  Trigonometric Function : Trigonometry  Operator=cos
  Trigonometric Function2 : Trigonometry
  E : Outport
  wires:
  Trigonometric Function/1 -> Gain/1
  Trigonometric Function2/1 -> Gain2/1
  beta/1 -> Trigonometric Function2/1, Trigonometric Function/1
  Gain/1 -> Sum/1
  Sum/1 -> E/1
  Gain2/1 -> Sum/2

== system matrix6_drive/Object/F(q,q dot)/F(alpha,beta) ==
  q : Inport
  Constant : Constant  Value=F1
  Constant1 : Constant  Value=D1
  D(beta) : Subsystem
  Demux : Demux  Outputs=2
  F(beta) : Subsystem
  Product : Product
  Product1 : Product
  Sum : Sum
  Sum1 : Sum  Inputs=|++
  Sum2 : Sum  Inputs=|++
  Trigonometric Function : Trigonometry  Operator=cos
  Trigonometric Function2 : Trigonometry
  F(q) : Outport
  wires:
  Trigonometric Function2/1 -> Product1/1
  Product1/1 -> Sum/2
  Trigonometric Function/1 -> Product/1
  Product/1 -> Sum/1
  Demux/1 -> Trigonometric Function2/1, Trigonometric Function/1
  Sum/1 -> F(q)/1
  F(beta)/1(F) -> Sum1/1
  Constant/1 -> Sum1/2
  Sum1/1 -> Product/2
  Demux/2 -> D(beta)/1(beta), F(beta)/1(beta)
  D(beta)/1(D) -> Sum2/1
  Constant1/1 -> Sum2/2
  Sum2/1 -> Product1/2
  q/1 -> Demux/1

== system matrix6_drive/Object/F(q,q dot)/F(beta) ==
  beta : Inport
  Gain : Gain  Gain=F2
  Gain1 : Gain  Gain=2
  Gain2 : Gain  Gain=(A2-B2)/2
  Sum : Sum  Inputs=+-
  Trigonometric Function : Trigonometry  Operator=cos
  Trigonometric Function2 : Trigonometry
  F : Outport
  wires:
  Trigonometric Function/1 -> Gain/1
  Trigonometric Function2/1 -> Gain2/1
  beta/1 -> Trigonometric Function/1, Gain1/1
  Gain/1 -> Sum/1
  Sum/1 -> F/1
  Gain2/1 -> Sum/2
  Gain1/1 -> Trigonometric Function2/1

== system matrix6_drive/Object/W(t,q)/w alpha (t, q)  ==
  Omega : Inport
  Omega dot : Inport  Port=2
  q : Inport  Port=3
  Sum : Sum  Inputs=|++
  bracket1 : Subsystem
  bracket2 : Subsystem
  w alpha : Outport
  wires:
  Omega dot/1 -> bracket1/1(Omega dot)
  q/1 -> bracket2/2(q), bracket1/2(q)
  Omega/1 -> bracket2/1(Omega)
  bracket1/1(Out1) -> Sum/1
  bracket2/1(Out1) -> Sum/2
  Sum/1 -> w alpha/1

== system matrix6_drive/Object/W(t,q)/w beta (t, q) ==
  Omega : Inport
  Omega dot : Inport  Port=2
  q : Inport  Port=3
  Gain : Gain  Gain=1/2
  Sum : Sum  Inputs=|+-
  bracket1 : Subsystem
  bracket2 : Subsystem
  w alpha : Outport
  wires:
  Sum/1 -> w alpha/1
  bracket2/1(Out1) -> Gain/1
  bracket1/1(Out1) -> Sum/1
  Omega/1 -> bracket2/1(Omega)
  q/1 -> bracket1/2(q), bracket2/2(q)
  Omega dot/1 -> bracket1/1(Omega dot)
  Gain/1 -> Sum/2

== system matrix6_drive/Drive/Привод/EM torque/Subsystem ==
  electrical angle : Inport
  phase : Inport  Port=2
  Sum1 : Sum  Inputs=++|
  Trigonometric Function1 : Trigonometry  Operator=cos
  Out1 : Outport
  wires:
  electrical angle/1 -> Sum1/1
  Sum1/1 -> Trigonometric Function1/1
  phase/1 -> Sum1/2
  Trigonometric Function1/1 -> Out1/1

== system matrix6_drive/Drive/Привод/EM torque/Subsystem1 ==
  electrical angle : Inport
  phase : Inport  Port=2
  Sum1 : Sum  Inputs=++|
  Trigonometric Function1 : Trigonometry  Operator=cos
  Out1 : Outport
  wires:
  electrical angle/1 -> Sum1/1
  Sum1/1 -> Trigonometric Function1/1
  phase/1 -> Sum1/2
  Trigonometric Function1/1 -> Out1/1

== system matrix6_drive/Drive/Привод/EM torque/Subsystem2 ==
  electrical angle : Inport
  phase : Inport  Port=2
  Sum1 : Sum  Inputs=++|
  Trigonometric Function1 : Trigonometry  Operator=cos
  Out1 : Outport
  wires:
  electrical angle/1 -> Sum1/1
  Sum1/1 -> Trigonometric Function1/1
  phase/1 -> Sum1/2
  Trigonometric Function1/1 -> Out1/1

== system matrix6_drive/Drive/Привод/EMFa/Subsystem ==
  electrical angle : Inport
  phase : Inport  Port=2
  Sum1 : Sum  Inputs=++|
  Trigonometric Function1 : Trigonometry  Operator=cos
  Out1 : Outport
  wires:
  electrical angle/1 -> Sum1/1
  Sum1/1 -> Trigonometric Function1/1
  phase/1 -> Sum1/2
  Trigonometric Function1/1 -> Out1/1

== system matrix6_drive/Drive/Привод1/EM torque/Subsystem ==
  electrical angle : Inport
  phase : Inport  Port=2
  Sum1 : Sum  Inputs=++|
  Trigonometric Function1 : Trigonometry  Operator=cos
  Out1 : Outport
  wires:
  Trigonometric Function1/1 -> Out1/1
  phase/1 -> Sum1/2
  Sum1/1 -> Trigonometric Function1/1
  electrical angle/1 -> Sum1/1

== system matrix6_drive/Drive/Привод1/EM torque/Subsystem1 ==
  electrical angle : Inport
  phase : Inport  Port=2
  Sum1 : Sum  Inputs=++|
  Trigonometric Function1 : Trigonometry  Operator=cos
  Out1 : Outport
  wires:
  Trigonometric Function1/1 -> Out1/1
  phase/1 -> Sum1/2
  Sum1/1 -> Trigonometric Function1/1
  electrical angle/1 -> Sum1/1

== system matrix6_drive/Drive/Привод1/EM torque/Subsystem2 ==
  electrical angle : Inport
  phase : Inport  Port=2
  Sum1 : Sum  Inputs=++|
  Trigonometric Function1 : Trigonometry  Operator=cos
  Out1 : Outport
  wires:
  Trigonometric Function1/1 -> Out1/1
  phase/1 -> Sum1/2
  Sum1/1 -> Trigonometric Function1/1
  electrical angle/1 -> Sum1/1

== system matrix6_drive/Drive/Привод1/EMFa/Subsystem ==
  electrical angle : Inport
  phase : Inport  Port=2
  Sum1 : Sum  Inputs=++|
  Trigonometric Function1 : Trigonometry  Operator=cos
  Out1 : Outport
  wires:
  Trigonometric Function1/1 -> Out1/1
  phase/1 -> Sum1/2
  Sum1/1 -> Trigonometric Function1/1
  electrical angle/1 -> Sum1/1

== system matrix6_drive/Object/B(t,q)/b(t,alpha,beta)/A2(beta) ==
  beta : Inport
  Gain : Gain  Gain=(A2-B2)/2
  Gain1 : Gain  Gain=2
  Gain2 : Gain  Gain=F2
  Sum : Sum
  Trigonometric Function : Trigonometry  Operator=cos
  Trigonometric Function2 : Trigonometry
  A2 : Outport
  wires:
  Trigonometric Function/1 -> Gain/1
  Trigonometric Function2/1 -> Gain2/1
  beta/1 -> Gain1/1
  Gain/1 -> Sum/1
  Sum/1 -> A2/1
  Gain2/1 -> Sum/2
  Gain1/1 -> Trigonometric Function2/1, Trigonometric Function/1

== system matrix6_drive/Object/B(t,q)/b(t,alpha,beta)/E(beta) ==
  beta : Inport
  Gain : Gain  Gain=E2
  Gain2 : Gain  Gain=D2
  Sum : Sum  Inputs=+-
  Trigonometric Function : Trigonometry  Operator=cos
  Trigonometric Function2 : Trigonometry
  E : Outport
  wires:
  Trigonometric Function/1 -> Gain/1
  Trigonometric Function2/1 -> Gain2/1
  beta/1 -> Trigonometric Function2/1, Trigonometric Function/1
  Gain/1 -> Sum/1
  Sum/1 -> E/1
  Gain2/1 -> Sum/2

== system matrix6_drive/Object/B(t,q)/b(t,alpha,beta)/F(beta) ==
  beta : Inport
  Gain : Gain  Gain=F2
  Gain1 : Gain  Gain=2
  Gain2 : Gain  Gain=(A2-B2)/2
  Sum : Sum  Inputs=+-
  Trigonometric Function : Trigonometry  Operator=cos
  Trigonometric Function2 : Trigonometry
  F : Outport
  wires:
  Trigonometric Function/1 -> Gain/1
  Trigonometric Function2/1 -> Gain2/1
  beta/1 -> Trigonometric Function/1, Gain1/1
  Gain/1 -> Sum/1
  Sum/1 -> F/1
  Gain2/1 -> Sum/2
  Gain1/1 -> Trigonometric Function2/1

== system matrix6_drive/Object/F(q,q dot)/F(alpha,beta)/D(beta) ==
  beta : Inport
  Gain : Gain  Gain=D2
  Gain2 : Gain  Gain=E2
  Sum : Sum
  Trigonometric Function : Trigonometry  Operator=cos
  Trigonometric Function2 : Trigonometry
  D : Outport
  wires:
  Trigonometric Function/1 -> Gain/1
  Trigonometric Function2/1 -> Gain2/1
  beta/1 -> Trigonometric Function2/1, Trigonometric Function/1
  Gain/1 -> Sum/1
  Sum/1 -> D/1
  Gain2/1 -> Sum/2

== system matrix6_drive/Object/F(q,q dot)/F(alpha,beta)/F(beta) ==
  beta : Inport
  Gain : Gain  Gain=F2
  Gain1 : Gain  Gain=2
  Gain2 : Gain  Gain=(A2-B2)/2
  Sum : Sum  Inputs=+-
  Trigonometric Function : Trigonometry  Operator=cos
  Trigonometric Function2 : Trigonometry
  F : Outport
  wires:
  Trigonometric Function/1 -> Gain/1
  Trigonometric Function2/1 -> Gain2/1
  beta/1 -> Trigonometric Function/1, Gain1/1
  Gain/1 -> Sum/1
  Sum/1 -> F/1
  Gain2/1 -> Sum/2
  Gain1/1 -> Trigonometric Function2/1

== system matrix6_drive/Object/W(t,q)/w alpha (t, q) /bracket1 ==
  Omega dot : Inport
  q : Inport  Port=2
  B(beta) : Subsystem
  Constant7 : Constant  Value=B1
  D(alpha,beta) : Subsystem
  Demux : Demux  Outputs=3
  Demux1 : Demux  Outputs=2
  F(alpha,beta) : Subsystem
  Product : Product
  Product1 : Product
  Product2 : Product
  Sum : Sum  Inputs=|++
  Sum1 : Sum  Inputs=-+-
  Out1 : Outport
  wires:
  Demux/2 -> Product1/1
  F(alpha,beta)/1(F(q)) -> Product/2
  Demux/1 -> Product/1
  Product/1 -> Sum1/1
  D(alpha,beta)/1(D(q)) -> Product2/2
  Demux1/2 -> B(beta)/1(beta)
  Product2/1 -> Sum1/3
  Product1/1 -> Sum1/2
  B(beta)/1(B) -> Sum/1
  q/1 -> D(alpha,beta)/1(q), Demux1/1, F(alpha,beta)/1(q)
  Sum/1 -> Product1/2  "a11"
  Demux/3 -> Product2/1
  Constant7/1 -> Sum/2
  Omega dot/1 -> Demux/1
  Sum1/1 -> Out1/1

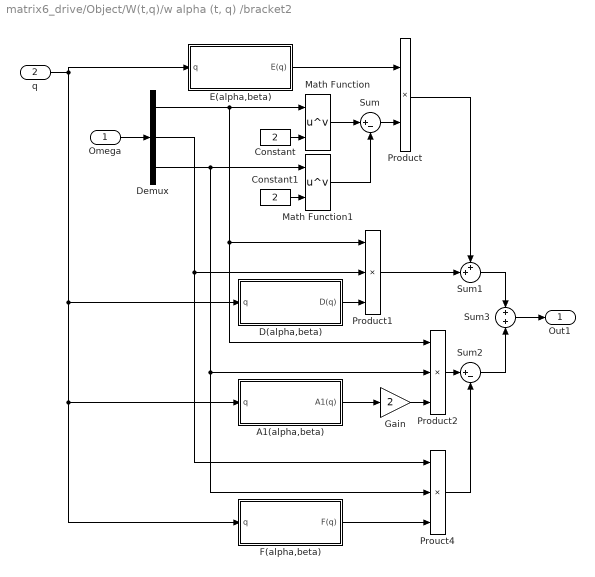
== system matrix6_drive/Object/W(t,q)/w alpha (t, q) /bracket2 ==
  Omega : Inport
  q : Inport  Port=2
  A1(alpha,beta) : Subsystem
  Constant : Constant  Value=2
  Constant1 : Constant  Value=2
  D(alpha,beta) : Subsystem
  Demux : Demux  Outputs=3
  E(alpha,beta) : Subsystem
  F(alpha,beta) : Subsystem
  Gain : Gain  Gain=2
  Math Function : Math  Operator=pow  SaturateOnIntegerOverflow=on
  Math Function1 : Math  Operator=pow  SaturateOnIntegerOverflow=on
  Product : Product
  Product1 : Product  Inputs=3
  Product2 : Product  Inputs=3
  Prouct4 : Product  Inputs=3
  Sum : Sum  Inputs=|+-
  Sum1 : Sum  Inputs=++|
  Sum2 : Sum  Inputs=|+-
  Sum3 : Sum
  Out1 : Outport
  wires:
  Omega/1 -> Demux/1
  Constant/1 -> Math Function/2
  Demux/1 -> Product2/1, Product1/1, Math Function/1
  Constant1/1 -> Math Function1/2
  Math Function/1 -> Sum/1
  Math Function1/1 -> Sum/2
  E(alpha,beta)/1(E(q)) -> Product/1
  Sum/1 -> Product/2
  q/1 -> F(alpha,beta)/1(q), A1(alpha,beta)/1(q), D(alpha,beta)/1(q), E(alpha,beta)/1(q)
  Demux/2 -> Prouct4/1, Product1/2
  D(alpha,beta)/1(D(q)) -> Product1/3
  A1(alpha,beta)/1(A1(q)) -> Gain/1
  Gain/1 -> Product2/3
  F(alpha,beta)/1(F(q)) -> Prouct4/3
  Demux/3 -> Prouct4/2, Product2/2, Math Function1/1
  Product/1 -> Sum1/1
  Product1/1 -> Sum1/2
  Prouct4/1 -> Sum2/2
  Product2/1 -> Sum2/1
  Sum1/1 -> Sum3/1
  Sum2/1 -> Sum3/2
  Sum3/1 -> Out1/1

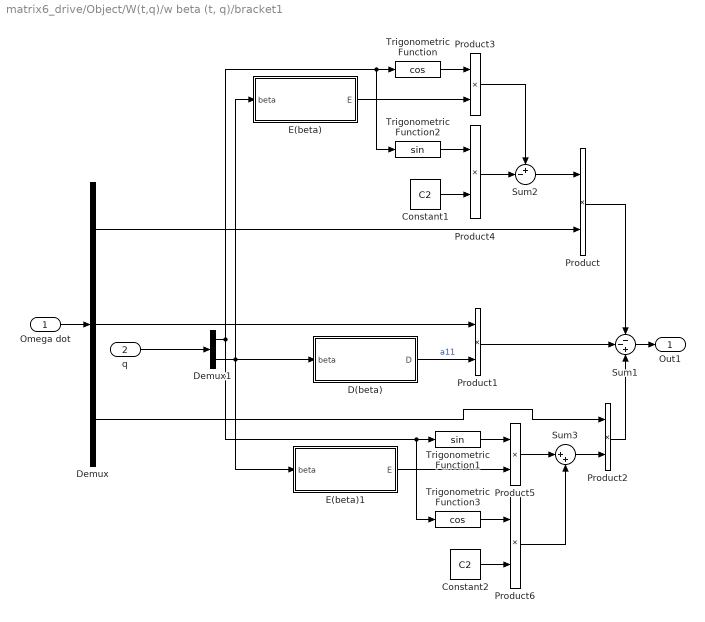
== system matrix6_drive/Object/W(t,q)/w beta (t, q)/bracket1 ==
  Omega dot : Inport
  q : Inport  Port=2
  Constant1 : Constant  Value=C2
  Constant2 : Constant  Value=C2
  D(beta) : Subsystem
  Demux : Demux  Outputs=3
  Demux1 : Demux  Outputs=2
  E(beta) : Subsystem
  E(beta)1 : Subsystem
  Product{,1..6} (7 alike) : Product
  Sum1 : Sum  Inputs=--+
  Sum2 : Sum  Inputs=+-|
  Sum3 : Sum  Inputs=|++
  Trigonometric Function : Trigonometry  Operator=cos
  Trigonometric Function1 : Trigonometry
  Trigonometric Function2 : Trigonometry
  Trigonometric Function3 : Trigonometry  Operator=cos
  Out1 : Outport
  wires:
  Sum1/1 -> Out1/1
  Omega dot/1 -> Demux/1
  Demux/3 -> Product2/1
  D(beta)/1(D) -> Product1/2  "a11"
  q/1 -> Demux1/1
  Product1/1 -> Sum1/2
  Product2/1 -> Sum1/3
  Demux1/2 -> E(beta)1/1(beta), D(beta)/1(beta), E(beta)/1(beta)
  Product/1 -> Sum1/1
  Demux/1 -> Product/2
  Sum2/1 -> Product/1
  Demux/2 -> Product1/1
  Constant1/1 -> Product4/2
  Trigonometric Function/1 -> Product3/1
  Product4/1 -> Sum2/2
  Trigonometric Function2/1 -> Product4/1
  E(beta)/1(E) -> Product3/2
  Product3/1 -> Sum2/1
  Constant2/1 -> Product6/2
  Product5/1 -> Sum3/1
  Trigonometric Function3/1 -> Product6/1
  E(beta)1/1(E) -> Product5/2
  Sum3/1 -> Product2/2
  Trigonometric Function1/1 -> Product5/1
  Product6/1 -> Sum3/2
  Demux1/1 -> Trigonometric Function/1, Trigonometric Function2/1, Trigonometric Function1/1, Trigonometric Function3/1

== system matrix6_drive/Object/W(t,q)/w beta (t, q)/bracket2 ==
  Omega : Inport
  q : Inport  Port=2
  Demux : Demux  Outputs=3
  Gain4 : Gain  Gain=2
  Product13 : Product
  Product14 : Product
  Product15 : Product
  Subsystem : Subsystem
  Subsystem1 : Subsystem
  Subsystem2 : Subsystem
  Subsystem3 : Subsystem
  Sum1 : Sum  Inputs=++|
  Sum8 : Sum  Inputs=+--
  Out1 : Outport
  wires:
  Demux/3 -> Product15/2, Product14/2
  Demux/2 -> Product15/1, Product13/2
  q/1 -> Subsystem/2(q), Subsystem3/1(q), Subsystem2/1(q), Subsystem1/1(q)
  Demux/1 -> Product14/1, Product13/1
  Omega/1 -> Subsystem/1(Omega), Demux/1
  Sum8/1 -> Gain4/1
  Gain4/1 -> Sum1/2
  Subsystem/1(Out1) -> Sum1/1
  Product13/1 -> Subsystem1/2(omega x omega y)
  Product14/1 -> Subsystem2/2(omega x omega z)
  Product15/1 -> Subsystem3/2(omega y omega z)
  Subsystem1/1(Out1) -> Sum8/1
  Subsystem2/1(Out1) -> Sum8/2
  Subsystem3/1(Out1) -> Sum8/3
  Sum1/1 -> Out1/1

== system matrix6_drive/Object/W(t,q)/w alpha (t, q) /bracket1/B(beta) ==
  beta : Inport
  Constant3 : Constant  Value=2
  Constant4 : Constant  Value=2
  Gain : Gain  Gain=B2
  Gain1 : Gain  Gain=A2
  Gain2 : Gain  Gain=F2
  Gain3 : Gain  Gain=2
  Math Function : Math  Operator=pow  SaturateOnIntegerOverflow=on
  Math Function1 : Math  Operator=pow  SaturateOnIntegerOverflow=on
  Sum : Sum  Inputs=++-
  Trigonometric Function : Trigonometry  Operator=cos
  Trigonometric Function1 : Trigonometry
  Trigonometric Function2 : Trigonometry
  B : Outport
  wires:
  beta/1 -> Gain3/1, Trigonometric Function1/1, Trigonometric Function/1
  Constant3/1 -> Math Function/2
  Trigonometric Function/1 -> Math Function/1
  Math Function/1 -> Gain/1
  Trigonometric Function1/1 -> Math Function1/1
  Math Function1/1 -> Gain1/1
  Constant4/1 -> Math Function1/2
  Trigonometric Function2/1 -> Gain2/1
  Gain3/1 -> Trigonometric Function2/1
  Gain1/1 -> Sum/2
  Gain/1 -> Sum/1
  Gain2/1 -> Sum/3
  Sum/1 -> B/1

== system matrix6_drive/Object/W(t,q)/w alpha (t, q) /bracket1/D(alpha,beta) ==
  q : Inport
  Constant : Constant  Value=F1
  Constant1 : Constant  Value=D1
  D(beta) : Subsystem
  Demux : Demux  Outputs=2
  F(beta) : Subsystem
  Product : Product
  Product1 : Product
  Sum : Sum  Inputs=-+
  Sum1 : Sum  Inputs=|++
  Sum2 : Sum  Inputs=|++
  Trigonometric Function : Trigonometry
  Trigonometric Function2 : Trigonometry  Operator=cos
  D(q) : Outport
  wires:
  Trigonometric Function2/1 -> Product1/1
  Product1/1 -> Sum/2
  Trigonometric Function/1 -> Product/1
  Product/1 -> Sum/1
  Demux/1 -> Trigonometric Function2/1, Trigonometric Function/1
  Sum/1 -> D(q)/1
  F(beta)/1(F) -> Sum1/1
  Constant/1 -> Sum1/2
  Sum1/1 -> Product/2
  Demux/2 -> D(beta)/1(beta), F(beta)/1(beta)
  D(beta)/1(D) -> Sum2/1
  Constant1/1 -> Sum2/2
  Sum2/1 -> Product1/2
  q/1 -> Demux/1

== system matrix6_drive/Object/W(t,q)/w alpha (t, q) /bracket1/F(alpha,beta) ==
  q : Inport
  Constant : Constant  Value=F1
  Constant1 : Constant  Value=D1
  D(beta) : Subsystem
  Demux : Demux  Outputs=2
  F(beta) : Subsystem
  Product : Product
  Product1 : Product
  Sum : Sum
  Sum1 : Sum  Inputs=|++
  Sum2 : Sum  Inputs=|++
  Trigonometric Function : Trigonometry  Operator=cos
  Trigonometric Function2 : Trigonometry
  F(q) : Outport
  wires:
  Trigonometric Function2/1 -> Product1/1
  Product1/1 -> Sum/2
  Trigonometric Function/1 -> Product/1
  Product/1 -> Sum/1
  Demux/1 -> Trigonometric Function2/1, Trigonometric Function/1
  Sum/1 -> F(q)/1
  F(beta)/1(F) -> Sum1/1
  Constant/1 -> Sum1/2
  Sum1/1 -> Product/2
  Demux/2 -> D(beta)/1(beta), F(beta)/1(beta)
  D(beta)/1(D) -> Sum2/1
  Constant1/1 -> Sum2/2
  Sum2/1 -> Product1/2
  q/1 -> Demux/1
